simulink model "validate_vapour_pressure_mdl"  (Simulink 7.6)
settings: Solver=FixedStepDiscrete  StartTime=0.0  StopTime=1  FixedStep=1  RelTol=1e-3
values from neighbouring files (symbols this model uses):
  fmix = mix(n)    [verification_density.m]    (also in verification_fluidproperty.m; verification_heat_capacity.m; verification_kinematic_viscosity.m; verification_thermal_conductivity.m)
  press = p(m)    [verification_density.m]    (also in verification_fluidproperty.m; verification_heat_capacity.m; verification_kinematic_viscosity.m; verification_thermal_conductivity.m)
undefined symbols (not defined in the file or in its folder): fluid
libraries: carnot x1
settings Model: Creator=drhf  LastModifiedBy=drhf
settings DataIOCC: SaveTime=off  ReturnWorkspaceOutputs=on  OutputSaveName=rho2

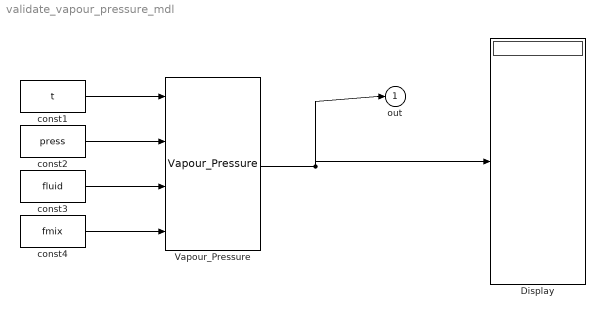
== system validate_vapour_pressure_mdl ==
  Display : Display
  Vapour_Pressure : carnot/Basic/Material_Properties/Vapour_Pressure  SystemSampleTime=-1
  const1 : Constant  Value=t
  const2 : Constant  Value=press
  const3 : Constant  Value=fluid
  const4 : Constant  Value=fmix
  out : Outport  InitialOutput=0
  wires:
  Vapour_Pressure/1 -> Display/1, out/1
  const1/1 -> Vapour_Pressure/1
  const2/1 -> Vapour_Pressure/2
  const3/1 -> Vapour_Pressure/3
  const4/1 -> Vapour_Pressure/4
